simulink model "sim2_ester"  (R2025b)
settings: Solver=FixedStepAuto  StartTime=0.0  StopTime=10.0  FixedStep=0.0001  RelTol=1e-3
values from neighbouring files (symbols this model uses):
  Beq = B_eq_est    [lab2_directDigitalDesign_ester.m]    (also in lab2_ssCT_ester.m; lab2_ssDT_ester.m)
  Dd = Dd_options(method_choice,:)    [lab2_pidDT_ester.m]
  Jeq = J_eq_est    [lab2_directDigitalDesign_ester.m]    (also in lab2_ssCT_ester.m; lab2_ssDT_ester.m)
  Ki = Ke(1)    [lab2_directDigitalDesign_ester.m]    (also in lab2_ssCT_ester.m = 0; lab2_ssDT_ester.m = 0)
  Kw = 5/0.15    (= 33.3333333333)    [lab2_pidDT_ester.m]
  method_choice = input('Choose discretization method (1 = B. Euler, 2 = F. Euler, 3 = Tustin): ')    [lab2_pidDT_ester.m]    (also in lab2_ssDT_ester.m = input('Choose discretization method (1 = F. Euler, 2 = B. Eu)
  Nd = Nd_options(method_choice,:)    [lab2_pidDT_ester.m]
  step_amplitude = 50    [lab2_directDigitalDesign_ester.m]    (also in lab2_pidDT_ester.m = 360; lab2_ssDT_ester.m)
  T = input('Select sample time (0.001, 0.01, 0.05) [s]: ')    [lab2_directDigitalDesign_ester.m]    (also in lab2_pidDT_ester.m; lab2_ssCT_ester.m = sampleTime_options(1); lab2_ssDT_ester.m)
undefined symbols (not defined in the file or in its folder): daq, DiscIntNeverNeededParam, drv, gbox, Kd, Kp, mot, pulse2deg, rads2rpm, Req, tau_sf_est
settings Model: Creator=ester  LastModifiedBy=ester
settings DebuggingCC: AlgebraicLoopMsg=none

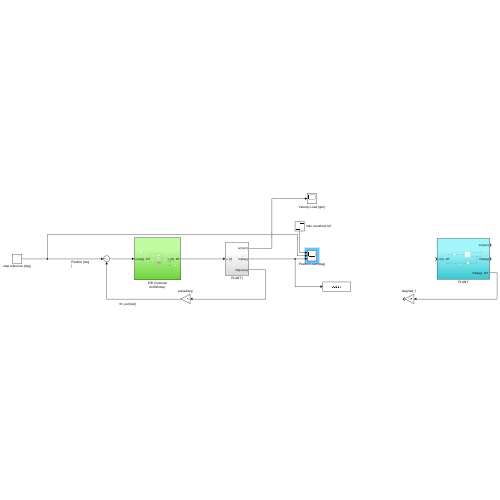
[thumbnail: Simulink's stored preview of the top-level diagram]
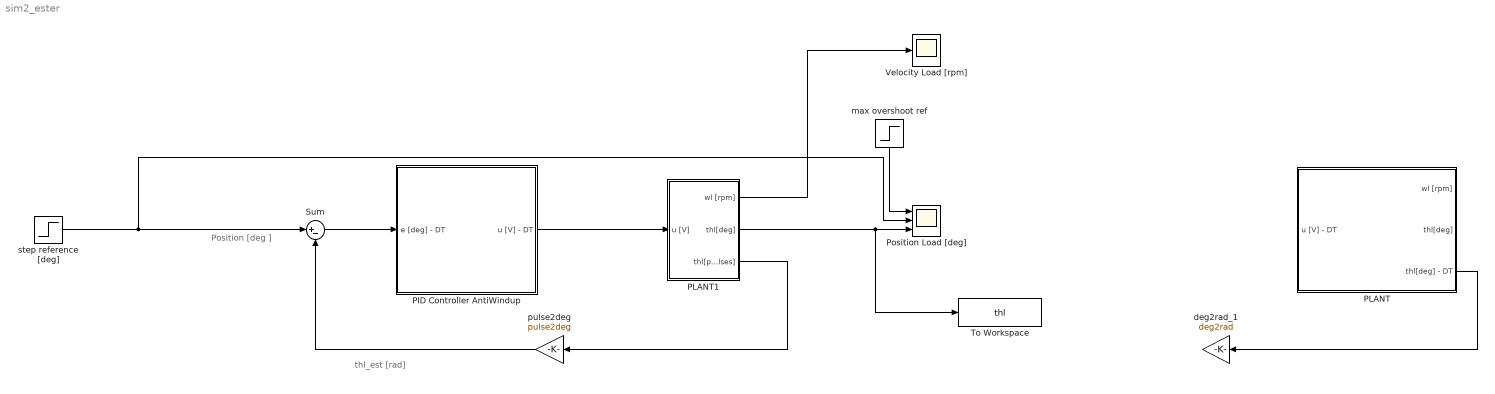
== system sim2_ester ==
  note: Position [deg
      | ]
  note: thl_est [rad]
  "PID Controller AntiWindup " : Subsystem
  PLANT : Subsystem
  PLANT1 : Subsystem
  Position Load [deg] : Scope  NumInputPorts=3
      settings: ActiveDisplayYMinimum=359.33333333333337  ActiveDisplayYMaximum=412.50000000000006
  Sum : Sum  Inputs=|+-
  To Workspace : ToWorkspace  VariableName=thl  SampleTime=T
  Velocity Load [rpm] : Scope
      settings: ActiveDisplayYMinimum=418.8599  ActiveDisplayYMaximum=462.8738
  deg2rad_1 : Gain  Gain=deg2rad
  max overshoot ref : Step  Time=0  After=step_amplitude*1.1  SampleTime=T
  pulse2deg : Gain  Gain=pulse2deg
  step reference [deg] : Step  After=step_amplitude  SampleTime=T
  wires:
  "PID Controller AntiWindup "/1(u [V] - DT) -> PLANT1/1(u [V])
  Sum/1 -> "PID Controller AntiWindup "/1(e [deg] - DT)
  PLANT/3("thl[deg] - DT ") -> deg2rad_1/1
  pulse2deg/1 -> Sum/2
  PLANT1/1(wl [rpm]) -> Velocity Load [rpm]/1
  step reference [deg]/1 -> Sum/1, Position Load [deg]/2
  max overshoot ref/1 -> Position Load [deg]/1
  PLANT1/2(thl[deg]) -> To Workspace/1, Position Load [deg]/3
  PLANT1/3(thl[pulses]) -> pulse2deg/1

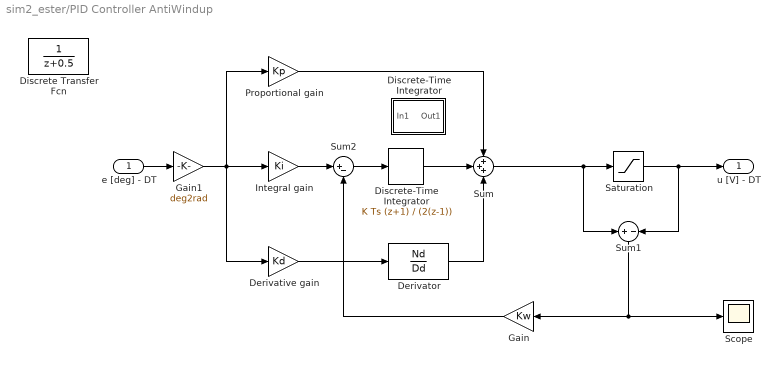
== system sim2_ester/PID Controller AntiWindup  ==
  e [deg] - DT : Inport
  Derivative gain : Gain  Gain=Kd
  "Derivator " : DiscreteTransferFcn  Numerator=Nd  Denominator=Dd
  Discrete Transfer Fcn : DiscreteTransferFcn
  "Discrete-Time Integrator " : DiscreteIntegrator  IntegratorMethod=Integration: Trapezoidal  SampleTime=T  ICPrevOutput=DiscIntNeverNeededParam  ICPrevScaledInput=DiscIntNeverNeededParam
  Discrete-Time Integrator : Subsystem
  Gain : Gain  Gain=Kw
  Gain1 : Gain  Gain=deg2rad
  "Integral gain " : Gain  Gain=Ki
  Proportional gain : Gain  Gain=Kp
  Saturation : Saturate  UpperLimit=daq.dac.fs  LowerLimit=-daq.dac.fs
  Scope : Scope
      settings: ActiveDisplayYMinimum=-13.77181697302583  ActiveDisplayYMaximum=123.94635275723249  DataLoggingVariableName=ScopeData2
  Sum : Sum  Inputs=+++
  Sum1 : Sum  Inputs=+|-
  Sum2 : Sum  Inputs=|+-
  u [V] - DT : Outport
  wires:
  "Derivator "/1 -> Sum/3
  e [deg] - DT/1 -> Gain1/1
  Proportional gain/1 -> Sum/1
  Derivative gain/1 -> "Derivator "/1
  Saturation/1 -> Sum1/2, u [V] - DT/1
  Sum1/1 -> Gain/1, Scope/1
  "Integral gain "/1 -> Sum2/1
  Gain/1 -> Sum2/2
  Sum/1 -> Sum1/1, Saturation/1
  Sum2/1 -> "Discrete-Time Integrator "/1
  "Discrete-Time Integrator "/1 -> Sum/2
  Gain1/1 -> Proportional gain/1, Derivative gain/1, "Integral gain "/1

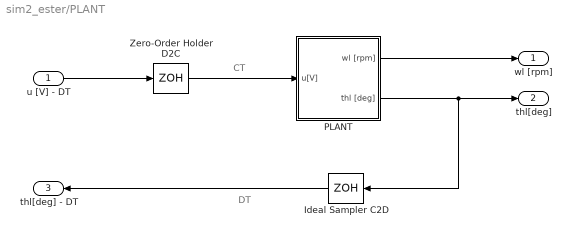
== system sim2_ester/PLANT ==
  note: DT
  note: CT
  u [V] - DT : Inport
  Ideal Sampler C2D : ZeroOrderHold  SampleTime=T
  PLANT : Subsystem
  Zero-Order Holder D2C : ZeroOrderHold  SampleTime=T
  wl [rpm] : Outport
  thl[deg] : Outport  Port=2
  "thl[deg] - DT " : Outport  Port=3
  wires:
  PLANT/2(thl [deg]) -> Ideal Sampler C2D/1, thl[deg]/1
  Ideal Sampler C2D/1 -> "thl[deg] - DT "/1
  u [V] - DT/1 -> Zero-Order Holder D2C/1
  PLANT/1(wl [rpm]) -> wl [rpm]/1
  Zero-Order Holder D2C/1 -> PLANT/1(u[V])

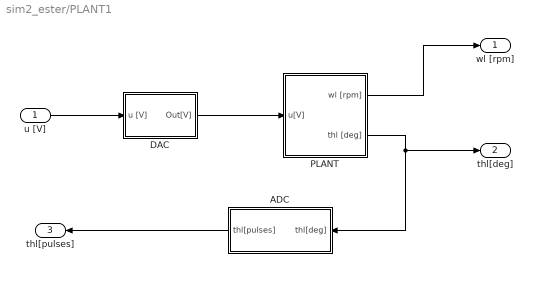
== system sim2_ester/PLANT1 ==
  u [V] : Inport
  ADC : Subsystem  TreatAsAtomicUnit=on
  DAC : Subsystem  TreatAsAtomicUnit=on
  PLANT : Subsystem
  wl [rpm] : Outport
  thl[deg] : Outport  Port=2
  thl[pulses] : Outport  Port=3
  wires:
  DAC/1(Out[V]) -> PLANT/1(u[V])
  PLANT/2(thl [deg]) -> thl[deg]/1, ADC/1(thl[deg])
  ADC/1(thl[pulses]) -> thl[pulses]/1
  u [V]/1 -> DAC/1(u [V])
  PLANT/1(wl [rpm]) -> wl [rpm]/1

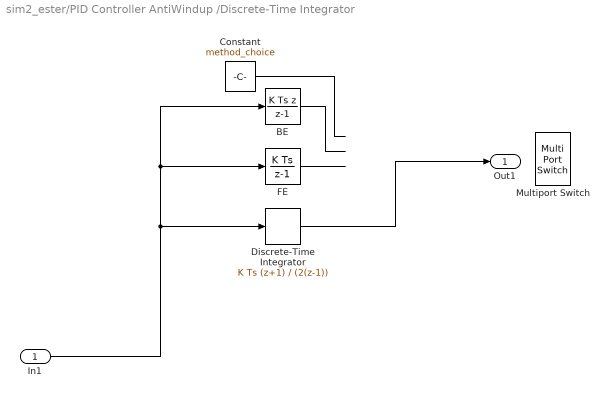
== system sim2_ester/PID Controller AntiWindup /Discrete-Time Integrator ==
  In1 : Inport
  BE : DiscreteIntegrator  IntegratorMethod=Integration: Backward Euler  SampleTime=T  ICPrevOutput=DiscIntNeverNeededParam  ICPrevScaledInput=DiscIntNeverNeededParam
  Constant : Constant  Value=method_choice
  "Discrete-Time Integrator " : DiscreteIntegrator  IntegratorMethod=Integration: Trapezoidal  SampleTime=T  ICPrevOutput=DiscIntNeverNeededParam  ICPrevScaledInput=DiscIntNeverNeededParam
  "FE " : DiscreteIntegrator  SampleTime=T  ICPrevOutput=DiscIntNeverNeededParam  ICPrevScaledInput=DiscIntNeverNeededParam
  Multiport Switch : MultiPortSwitch  SaturateOnIntegerOverflow=off  InputSameDT=off
  Out1 : Outport
  wires:
  In1/1 -> BE/1, "FE "/1, "Discrete-Time Integrator "/1
  Constant/1 -> ?
  "FE "/1 -> ?
  "Discrete-Time Integrator "/1 -> Out1/1
  BE/1 -> ?

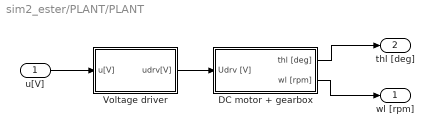
== system sim2_ester/PLANT/PLANT ==
  u[V] : Inport
  DC motor + gearbox : Subsystem
  Voltage driver : Subsystem  TreatAsAtomicUnit=on
  wl [rpm] : Outport
  thl [deg] : Outport  Port=2
  wires:
  Voltage driver/1(udrv[V]) -> DC motor + gearbox/1(Udrv [V])
  u[V]/1 -> Voltage driver/1(u[V])
  DC motor + gearbox/1(thl [deg]) -> thl [deg]/1
  DC motor + gearbox/2(wl [rpm]) -> wl [rpm]/1

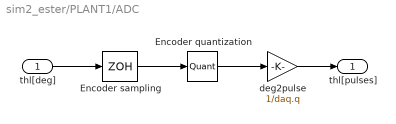
== system sim2_ester/PLANT1/ADC ==
  thl[deg] : Inport
  Encoder quantization : Quantizer  QuantizationInterval=daq.q
  Encoder sampling : ZeroOrderHold  SampleTime=daq.dac.Ts
  deg2pulse : Gain  Gain=1/daq.q
  thl[pulses] : Outport
  wires:
  Encoder quantization/1 -> deg2pulse/1
  thl[deg]/1 -> Encoder sampling/1
  Encoder sampling/1 -> Encoder quantization/1
  deg2pulse/1 -> thl[pulses]/1

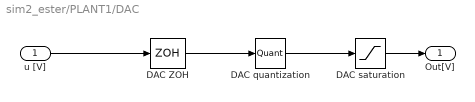
== system sim2_ester/PLANT1/DAC ==
  u [V] : Inport
  "DAC ZOH " : ZeroOrderHold  SampleTime=daq.dac.Ts
  DAC quantization : Quantizer  QuantizationInterval=daq.dac.q
  DAC saturation : Saturate  UpperLimit=daq.dac.fs  LowerLimit=-daq.dac.fs
  Out[V] : Outport
  wires:
  DAC quantization/1 -> DAC saturation/1
  u [V]/1 -> "DAC ZOH "/1
  "DAC ZOH "/1 -> DAC quantization/1
  DAC saturation/1 -> Out[V]/1

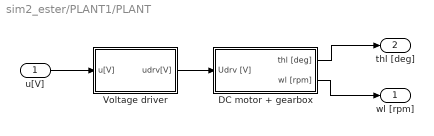
== system sim2_ester/PLANT1/PLANT ==
  u[V] : Inport
  DC motor + gearbox : Subsystem
  Voltage driver : Subsystem  TreatAsAtomicUnit=on
  wl [rpm] : Outport
  thl [deg] : Outport  Port=2
  wires:
  Voltage driver/1(udrv[V]) -> DC motor + gearbox/1(Udrv [V])
  u[V]/1 -> Voltage driver/1(u[V])
  DC motor + gearbox/1(thl [deg]) -> thl [deg]/1
  DC motor + gearbox/2(wl [rpm]) -> wl [rpm]/1

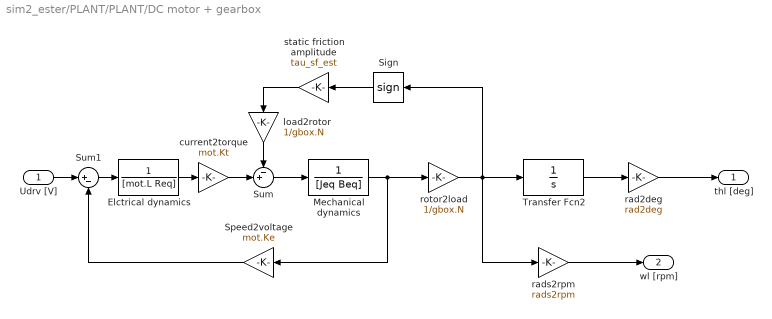
== system sim2_ester/PLANT/PLANT/DC motor + gearbox ==
  Udrv [V] : Inport
  Elctrical dynamics : TransferFcn  Denominator=[mot.L Req]
  Mechanical dynamics : TransferFcn  Denominator=[Jeq Beq]
  Sign : Signum  ZeroCross=off
  Speed2voltage : Gain  Gain=mot.Ke
  Sum : Sum  Inputs=-+|
  Sum1 : Sum  Inputs=|+-
  Transfer Fcn2 : TransferFcn  Denominator=[1 0]
  current2torque : Gain  Gain=mot.Kt
  load2rotor : Gain  Gain=1/gbox.N
  rad2deg : Gain  Gain=rad2deg
  rads2rpm : Gain  Gain=rads2rpm
  rotor2load : Gain  Gain=1/gbox.N
  static friction amplitude : Gain  Gain=tau_sf_est
  thl [deg] : Outport
  wl [rpm] : Outport  Port=2
  wires:
  rotor2load/1 -> Sign/1, rads2rpm/1, Transfer Fcn2/1
  Sign/1 -> static friction amplitude/1
  rads2rpm/1 -> wl [rpm]/1
  Sum/1 -> Mechanical dynamics/1
  Udrv [V]/1 -> Sum1/1
  static friction amplitude/1 -> load2rotor/1
  load2rotor/1 -> Sum/1
  Transfer Fcn2/1 -> rad2deg/1
  current2torque/1 -> Sum/2
  Speed2voltage/1 -> Sum1/2
  Mechanical dynamics/1 -> Speed2voltage/1, rotor2load/1
  Elctrical dynamics/1 -> current2torque/1
  Sum1/1 -> Elctrical dynamics/1
  rad2deg/1 -> thl [deg]/1

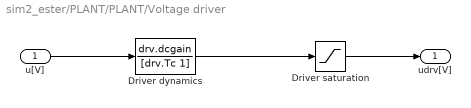
== system sim2_ester/PLANT/PLANT/Voltage driver ==
  u[V] : Inport
  Driver dynamics : TransferFcn  Numerator=drv.dcgain  Denominator=[drv.Tc 1]
  Driver saturation : Saturate  UpperLimit=drv.outmax  LowerLimit=-drv.outmax
  udrv[V] : Outport
  wires:
  Driver dynamics/1 -> Driver saturation/1
  u[V]/1 -> Driver dynamics/1
  Driver saturation/1 -> udrv[V]/1

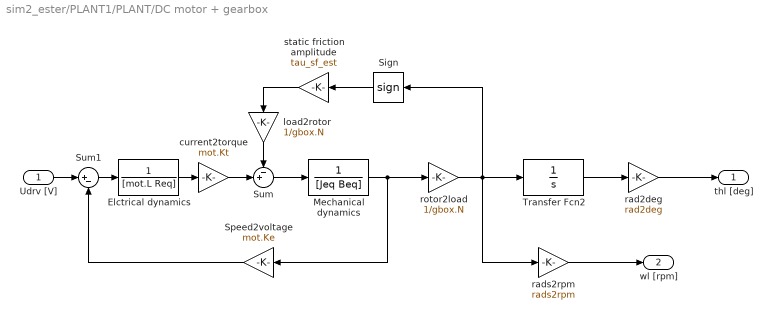
== system sim2_ester/PLANT1/PLANT/DC motor + gearbox ==
  Udrv [V] : Inport
  Elctrical dynamics : TransferFcn  Denominator=[mot.L Req]
  Mechanical dynamics : TransferFcn  Denominator=[Jeq Beq]
  Sign : Signum  ZeroCross=off
  Speed2voltage : Gain  Gain=mot.Ke
  Sum : Sum  Inputs=-+|
  Sum1 : Sum  Inputs=|+-
  Transfer Fcn2 : TransferFcn  Denominator=[1 0]
  current2torque : Gain  Gain=mot.Kt
  load2rotor : Gain  Gain=1/gbox.N
  rad2deg : Gain  Gain=rad2deg
  rads2rpm : Gain  Gain=rads2rpm
  rotor2load : Gain  Gain=1/gbox.N
  static friction amplitude : Gain  Gain=tau_sf_est
  thl [deg] : Outport
  wl [rpm] : Outport  Port=2
  wires:
  rotor2load/1 -> Sign/1, rads2rpm/1, Transfer Fcn2/1
  Sign/1 -> static friction amplitude/1
  rads2rpm/1 -> wl [rpm]/1
  Sum/1 -> Mechanical dynamics/1
  Udrv [V]/1 -> Sum1/1
  static friction amplitude/1 -> load2rotor/1
  load2rotor/1 -> Sum/1
  Transfer Fcn2/1 -> rad2deg/1
  current2torque/1 -> Sum/2
  Speed2voltage/1 -> Sum1/2
  Mechanical dynamics/1 -> Speed2voltage/1, rotor2load/1
  Elctrical dynamics/1 -> current2torque/1
  Sum1/1 -> Elctrical dynamics/1
  rad2deg/1 -> thl [deg]/1

== system sim2_ester/PLANT1/PLANT/Voltage driver ==
  u[V] : Inport
  Driver dynamics : TransferFcn  Numerator=drv.dcgain  Denominator=[drv.Tc 1]
  Driver saturation : Saturate  UpperLimit=drv.outmax  LowerLimit=-drv.outmax
  udrv[V] : Outport
  wires:
  Driver dynamics/1 -> Driver saturation/1
  u[V]/1 -> Driver dynamics/1
  Driver saturation/1 -> udrv[V]/1
